simulink model "sim_WAM_PBACDynamics"  (R2018b)
settings: Solver=FixedStepAuto  StartTime=0.0  StopTime=0  FixedStep=1e-3  RelTol=1e-3
values from neighbouring files (symbols this model uses):
  Cfcn = matlabFunction(Ctemp, 'vars', {q1, q2, q4, q1d, q2d, q4d})    [convertSymVarsTOfunctions.m]
  Ffcn = matlabFunction(Ftemp, 'vars', {q1d, q2d, q4d})    [convertSymVarsTOfunctions.m]
  Gamma = 5*eye(27)    [MAIN_FINAL.m]
  Gfcn = matlabFunction(Gtemp, 'vars', {q1, q2, q4})    [convertSymVarsTOfunctions.m]
  K = diag([10 30 10])    [MAIN_FINAL.m]    (also in PBMC_WAM.m = 10*diag([1 1 1]))
  Lambda = 5*eye(3)    [MAIN_FINAL.m]    (also in PBMC_WAM.m = 10*diag([1 1 1]))
  Mfcn = matlabFunction(Mtemp, 'vars', {q1, q2, q4})    [convertSymVarsTOfunctions.m]
  Q0 = [pi/4, pi/4, pi/4, pi/4, pi/4, pi/4]    [MAIN_FINAL.m]
  w = 2*pi/10    (= 0.628318530718)    [GetOptimalTrajectories.m]    (also in MAIN_FINAL.m = 1; MAIN_OptimalTrajectories.m; invDynWAM.m = 4; trajct1.mat)
  Yavfcn = matlabFunction(Yavtemp, 'vars', {q1, q2, q4, q1d, q2d, q4d, q1dd, q2dd, q4dd,                                                  v1, v2, v3, a1, a2, a3})    [convertSymVarsTOfunctions.m]
undefined symbols (not defined in the file or in its folder): getTHhat, PBAC_WAM, statederWAM
settings Model: Creator=Erivelton  LastModifiedBy=Erivelton

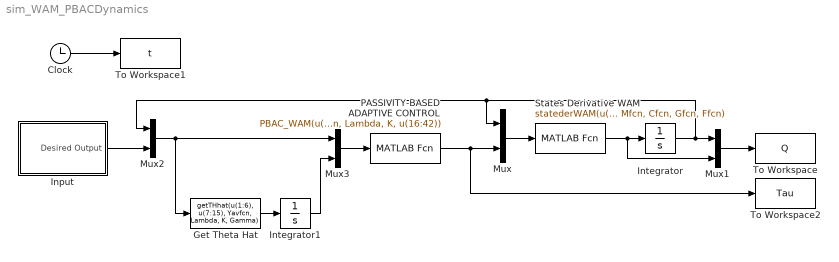
== system sim_WAM_PBACDynamics ==
  Clock : Clock
  Get Theta Hat : MATLABFcn  MATLABFcn=getTHhat(u(1:6), u(7:15), Yavfcn, Lambda, K, Gamma)  OutputDimensions=27
  Input : Subsystem
  Integrator : Integrator  InitialCondition=Q0
  Integrator1 : Integrator
  Mux{,1..3} (4 alike) : Mux  Inputs=2
  PASSIVITY-BASED ADAPTIVE CONTROL : MATLABFcn  MATLABFcn=PBAC_WAM(u(1:6), u(7:15), Yavfcn, Lambda, K, u(16:42))  OutputDimensions=3
  States Derivative WAM : MATLABFcn  MATLABFcn=statederWAM(u(1:6), u(7:9), Mfcn, Cfcn, Gfcn, Ffcn)  OutputDimensions=6
  To Workspace : ToWorkspace  VariableName=Q  SampleTime=-1
  To Workspace1 : ToWorkspace  VariableName=t  SampleTime=-1
  To Workspace2 : ToWorkspace  VariableName=Tau  SampleTime=-1
  wires:
  States Derivative WAM/1 -> Mux1/2, Integrator/1
  Mux/1 -> States Derivative WAM/1
  Integrator/1 -> Mux1/1, Mux/1, Mux2/1
  Clock/1 -> To Workspace1/1
  Mux1/1 -> To Workspace/1
  PASSIVITY-BASED ADAPTIVE CONTROL/1 -> To Workspace2/1, Mux/2
  Input/1(Desired Output) -> Mux2/2
  Mux2/1 -> Get Theta Hat/1, Mux3/1
  Mux3/1 -> PASSIVITY-BASED ADAPTIVE CONTROL/1
  Get Theta Hat/1 -> Integrator1/1
  Integrator1/1 -> Mux3/2

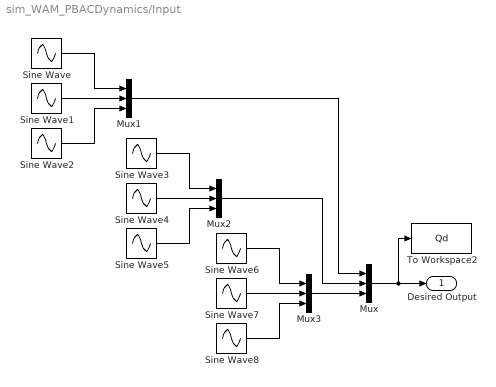
== system sim_WAM_PBACDynamics/Input ==
  Mux{,1..3} (4 alike) : Mux  Inputs=3
  Sine Wave : Sin  Frequency=w  SampleTime=0
  Sine Wave1 : Sin  Amplitude=w  Frequency=w  Phase=pi/2  SampleTime=0
  Sine Wave2 : Sin  Amplitude=-w*w  Frequency=w  SampleTime=0
  Sine Wave3 : Sin  Bias=-.5  Frequency=w  SampleTime=0
  Sine Wave4 : Sin  Amplitude=w  Frequency=w  Phase=pi/2  SampleTime=0
  Sine Wave5 : Sin  Amplitude=-w*w  Frequency=w  SampleTime=0
  Sine Wave6 : Sin  Amplitude=.75  Frequency=w  SampleTime=0
  Sine Wave7 : Sin  Amplitude=.75*w  Frequency=w  Phase=pi/2  SampleTime=0
  Sine Wave8 : Sin  Amplitude=-.75*w*w  Frequency=w  SampleTime=0
  To Workspace2 : ToWorkspace  VariableName=Qd  SampleTime=-1
  Desired Output : Outport
  wires:
  Mux/1 -> To Workspace2/1, Desired Output/1
  Mux3/1 -> Mux/3
  Mux2/1 -> Mux/2
  Mux1/1 -> Mux/1
  Sine Wave/1 -> Mux1/1
  Sine Wave1/1 -> Mux1/2
  Sine Wave2/1 -> Mux1/3
  Sine Wave5/1 -> Mux2/3
  Sine Wave4/1 -> Mux2/2
  Sine Wave3/1 -> Mux2/1
  Sine Wave8/1 -> Mux3/3
  Sine Wave7/1 -> Mux3/2
  Sine Wave6/1 -> Mux3/1
